simulink model "RPF_Mecanum_02"  (R2020b)
settings: Solver=VariableStepAuto  StartTime=0.0  StopTime=300  MaxStep=0.1  RelTol=1e-3
InitFcn:
  | RadioRueda = 0.05;
  | l1 = 0.15;
  | l2 = 0.15;
libraries: dspsigops x1, simulink x1
settings Model: Creator=rpiza  LastModifiedBy=Racarla

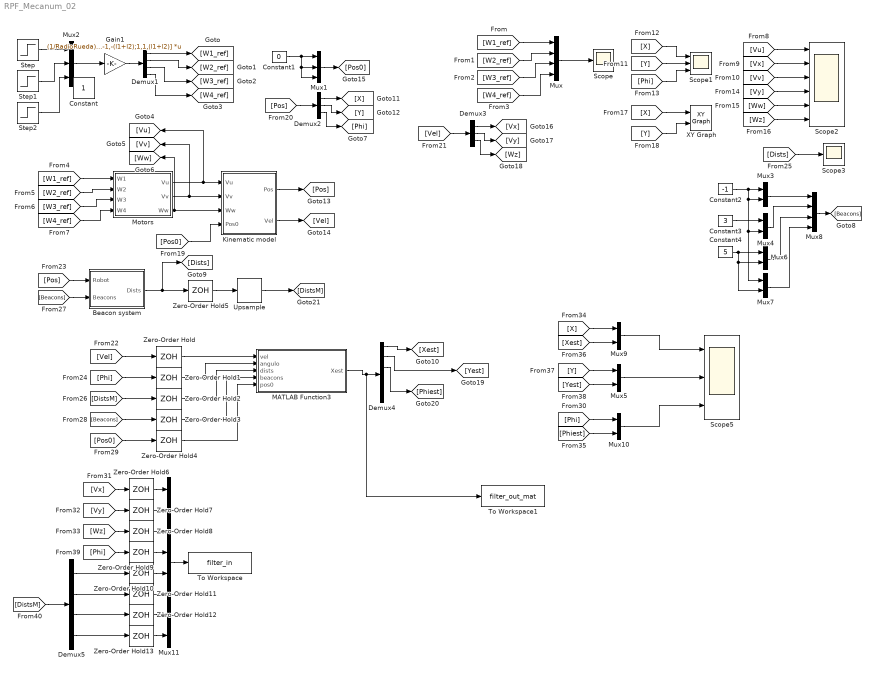
== system RPF_Mecanum_02 ==
  Beacon system : Subsystem
  Constant1 : Constant  Value=0
  Constant2 : Constant  Value=-1
  Constant3 : Constant  Value=3
  Constant4 : Constant  Value=5
  Demux1 : Demux
  Demux2 : Demux  Outputs=3
  Demux3 : Demux  Outputs=3
  Demux4 : Demux  Outputs=6
  Demux5 : Demux
  Gain1 : Gain  Gain=(1/RadioRueda)*[1,1,-(l1+l2); 1,-1,(l1+l2);1,-1,-(l1+l2);1,1,(l1+l2)]  Multiplication=Matrix(K*u) (u vector)
  Kinematic model : Subsystem
  MATLAB Function3 : MATLAB Function  TreatAsAtomicUnit=on
  Motors : Subsystem
  Mux : Mux
  Mux1 : Mux  Inputs=3
  Mux{3..7,9..10} (7 alike) : Mux  Inputs=2
  Mux11 : Mux  Inputs=8
  Mux2 : Mux  Inputs=3
  Mux8 : Mux
  Scope : Scope
  Scope1 : Scope  NumInputPorts=3
  Scope2 : Scope  NumInputPorts=6
  Scope3 : Scope
  Scope5 : Scope  NumInputPorts=3
  Step : Step  Time=0  After=0.1  SampleTime=0
  Step1 : Step  Time=5  Before=0.1  After=0  SampleTime=0
  Step2 : Step  Time=10  After=0.05  SampleTime=0
  To Workspace : ToWorkspace  VariableName=filter_in  SaveFormat=Timeseries  SampleTime=-1
  To Workspace1 : ToWorkspace  VariableName=filter_out_mat  SaveFormat=Timeseries  SampleTime=-1
  Upsample : dspsigops/Upsample  N=10  phase=0  RateOptions=Allow multirate processing  ic=0  mode=Unused parameter value
  XY Graph : simulink/Sinks/XY Graph  xmin=-1  xmax=3  ymin=-1  ymax=5  st=-1
  Zero-Order Hold{,1..4,6..13} (13 alike) : ZeroOrderHold  SampleTime=0.1
  Zero-Order Hold5 : ZeroOrderHold
  Constant : Constant  IOType=siggen
  wires:
  [W1_ref] -> Mux/1
  [W2_ref] -> Mux/2
  [W3_ref] -> Mux/3
  [W4_ref] -> Mux/4
  Mux/1 -> Scope/1
  [Vu] -> Scope2/1
  [Vx] -> Scope2/2
  [Vv] -> Scope2/3
  Mux2/1 -> Gain1/1
  [Vy] -> Scope2/4
  [Ww] -> Scope2/5
  [Wz] -> Scope2/6
  Gain1/1 -> Demux1/1
  Step/1 -> Mux2/1
  Step1/1 -> Mux2/2
  Step2/1 -> Mux2/3
  Demux1/1 -> [W1_ref]
  Demux1/4 -> [W4_ref]
  Demux1/3 -> [W3_ref]
  Demux1/2 -> [W2_ref]
  [Y] -> Scope1/2
  [X] -> Scope1/1
  [Phi] -> Scope1/3
  [X] -> XY Graph/1
  [Y] -> XY Graph/2
  Motors/1(Vu) -> [Vu], Kinematic model/1(Vu)
  Motors/2(Vv) -> [Vv], Kinematic model/2(Vv)
  Motors/3(Ww) -> Kinematic model/3(Ww), [Ww]
  [W1_ref] -> Motors/1(W1)
  [W2_ref] -> Motors/2(W2)
  [W3_ref] -> Motors/3(W3)
  [W4_ref] -> Motors/4(W4)
  Kinematic model/1(Pos) -> [Pos]
  Kinematic model/2(Vel) -> [Vel]
  Mux1/1 -> [Pos0]
  [Pos0] -> Kinematic model/4(Pos0)
  Constant1/1 -> Mux1/2, Mux1/3, Mux1/1
  [Pos] -> Demux2/1
  Demux2/1 -> [X]
  Demux2/2 -> [Y]
  Demux2/3 -> [Phi]
  Demux3/3 -> [Wz]
  Demux3/2 -> [Vy]
  Demux3/1 -> [Vx]
  [Vel] -> Demux3/1
  Constant2/1 -> Mux3/1, Mux4/2, Mux7/1, Mux3/2
  Mux3/1 -> Mux8/1
  Constant3/1 -> Mux4/1
  Mux4/1 -> Mux8/2
  Constant4/1 -> Mux6/1, Mux6/2, Mux7/2
  Mux6/1 -> Mux8/3
  Mux7/1 -> Mux8/4
  Mux8/1 -> [Beacons]
  [Pos] -> Beacon system/1(Robot)
  [Beacons] -> Beacon system/2(Beacons)
  Beacon system/1(Dists) -> Zero-Order Hold5/1, [Dists]
  [Dists] -> Scope3/1
  [Vel] -> Zero-Order Hold/1
  [Phi] -> Zero-Order Hold1/1
  [DistsM] -> Zero-Order Hold2/1
  Zero-Order Hold/1 -> MATLAB Function3/1(vel)
  MATLAB Function3/1(Xest) -> To Workspace1/1, Demux4/1
  [Beacons] -> Zero-Order Hold3/1
  Zero-Order Hold1/1 -> MATLAB Function3/2(angulo)
  Zero-Order Hold2/1 -> MATLAB Function3/3(dists)
  Zero-Order Hold3/1 -> MATLAB Function3/4(beacons)
  [Pos0] -> Zero-Order Hold4/1
  Zero-Order Hold4/1 -> MATLAB Function3/5(pos0)
  Mux5/1 -> Scope5/2
  [X] -> Mux9/1
  [Xest] -> Mux9/2
  Mux9/1 -> Scope5/1
  Demux4/1 -> [Xest]
  Demux4/2 -> [Yest]
  [Yest] -> Mux5/2
  [Y] -> Mux5/1
  [Phi] -> Mux10/1
  [Phiest] -> Mux10/2
  Demux4/3 -> [Phiest]
  Mux10/1 -> Scope5/3
  Zero-Order Hold5/1 -> Upsample/1
  Upsample/1 -> [DistsM]
  Mux11/1 -> To Workspace/1
  Zero-Order Hold6/1 -> Mux11/1
  Zero-Order Hold7/1 -> Mux11/2
  Zero-Order Hold8/1 -> Mux11/3
  Zero-Order Hold9/1 -> Mux11/4
  Zero-Order Hold10/1 -> Mux11/5
  Zero-Order Hold11/1 -> Mux11/6
  Zero-Order Hold12/1 -> Mux11/7
  Zero-Order Hold13/1 -> Mux11/8
  [Vx] -> Zero-Order Hold6/1
  [Vy] -> Zero-Order Hold7/1
  [Wz] -> Zero-Order Hold8/1
  [Phi] -> Zero-Order Hold9/1
  Demux5/1 -> Zero-Order Hold10/1
  Demux5/2 -> Zero-Order Hold11/1
  Demux5/3 -> Zero-Order Hold12/1
  Demux5/4 -> Zero-Order Hold13/1
  [DistsM] -> Demux5/1

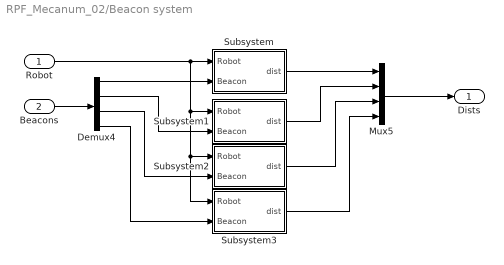
== system RPF_Mecanum_02/Beacon system ==
  Robot : Inport
  Beacons : Inport  Port=2
  Demux4 : Demux
  Mux5 : Mux
  Subsystem : Subsystem
  Subsystem1 : Subsystem
  Subsystem2 : Subsystem
  Subsystem3 : Subsystem
  Dists : Outport
  wires:
  Subsystem/1(dist) -> Mux5/1
  Mux5/1 -> Dists/1
  Robot/1 -> Subsystem/1(Robot), Subsystem1/1(Robot), Subsystem2/1(Robot), Subsystem3/1(Robot)
  Subsystem2/1(dist) -> Mux5/3
  Beacons/1 -> Demux4/1
  Subsystem1/1(dist) -> Mux5/2
  Subsystem3/1(dist) -> Mux5/4
  Demux4/1 -> Subsystem/2(Beacon)
  Demux4/2 -> Subsystem1/2(Beacon)
  Demux4/3 -> Subsystem2/2(Beacon)
  Demux4/4 -> Subsystem3/2(Beacon)

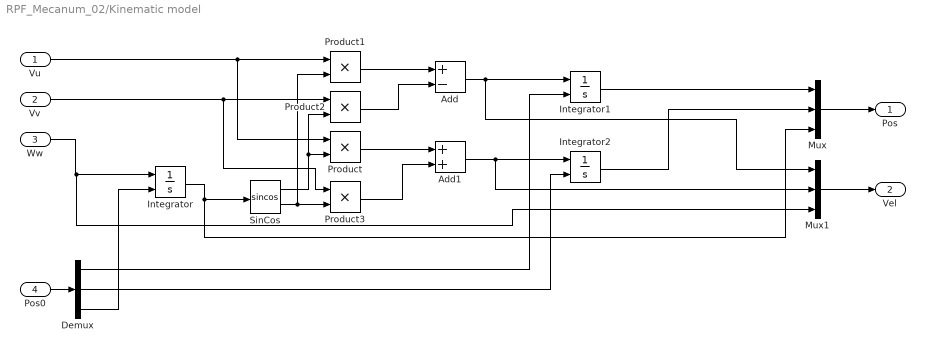
== system RPF_Mecanum_02/Kinematic model ==
  Vu : Inport
  Vv : Inport  Port=2
  Ww : Inport  Port=3
  Pos0 : Inport  Port=4
  Add : Sum  Inputs=+-
  Add1 : Sum
  Demux : Demux  Outputs=3
  Integrator : Integrator  InitialConditionSource=external
  Integrator1 : Integrator  InitialConditionSource=external
  Integrator2 : Integrator  InitialConditionSource=external
  Mux : Mux  Inputs=3
  Mux1 : Mux  Inputs=3
  Product{,1..3} (4 alike) : Product
  SinCos : Trigonometry  Operator=sincos
  Pos : Outport
  Vel : Outport  Port=2
  wires:
  Product/1 -> Add1/1
  SinCos/2 -> Product3/2, Product1/2
  Vv/1 -> Product3/1, Product2/1
  Add1/1 -> Mux1/2, Integrator2/1
  Ww/1 -> Mux1/3, Integrator/1
  Product2/1 -> Add/2
  Add/1 -> Mux1/1, Integrator1/1
  SinCos/1 -> Product2/2, Product/2
  Product3/1 -> Add1/2
  Integrator/1 -> Mux/3, SinCos/1
  Vu/1 -> Product/1, Product1/1
  Product1/1 -> Add/1
  Integrator2/1 -> Mux/2
  Integrator1/1 -> Mux/1
  Mux/1 -> Pos/1
  Mux1/1 -> Vel/1
  Pos0/1 -> Demux/1
  Demux/1 -> Integrator1/2
  Demux/2 -> Integrator2/2
  Demux/3 -> Integrator/2

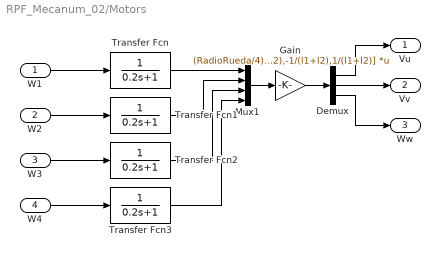
== system RPF_Mecanum_02/Motors ==
  W1 : Inport
  W2 : Inport  Port=2
  W3 : Inport  Port=3
  W4 : Inport  Port=4
  Demux : Demux  Outputs=3
  Gain : Gain  Gain=(RadioRueda/4)*[1,1,1,1;1,-1,-1,1;-1/(l1+l2),1/(l1+l2),-1/(l1+l2),1/(l1+l2)]  Multiplication=Matrix(K*u) (u vector)
  Mux1 : Mux
  Transfer Fcn{,1..3} (4 alike) : TransferFcn  Denominator=[0.2 1]
  Vu : Outport
  Vv : Outport  Port=2
  Ww : Outport  Port=3
  wires:
  Demux/2 -> Vv/1
  Mux1/1 -> Gain/1
  Transfer Fcn2/1 -> Mux1/3
  W4/1 -> Transfer Fcn3/1
  Transfer Fcn1/1 -> Mux1/2
  W3/1 -> Transfer Fcn2/1
  Transfer Fcn/1 -> Mux1/1
  Transfer Fcn3/1 -> Mux1/4
  Gain/1 -> Demux/1
  W2/1 -> Transfer Fcn1/1
  Demux/1 -> Vu/1
  W1/1 -> Transfer Fcn/1
  Demux/3 -> Ww/1

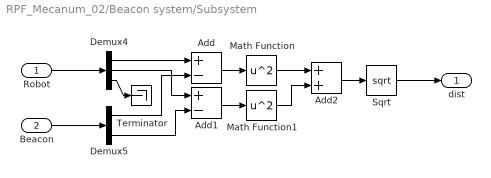
== system RPF_Mecanum_02/Beacon system/Subsystem ==
  Robot : Inport
  Beacon : Inport  Port=2
  Add : Sum  Inputs=+-
  Add1 : Sum  Inputs=+-
  Add2 : Sum
  Demux4 : Demux  Outputs=3
  Demux5 : Demux  Outputs=2
  Math Function : Math  Operator=square  SaturateOnIntegerOverflow=on
  Math Function1 : Math  Operator=square  SaturateOnIntegerOverflow=on
  Sqrt : Sqrt  SaturateOnIntegerOverflow=on
  Terminator : Terminator
  dist : Outport
  wires:
  Math Function/1 -> Add2/1
  Demux4/3 -> Terminator/1
  Add1/1 -> Math Function1/1
  Demux4/1 -> Add/1
  Math Function1/1 -> Add2/2
  Demux4/2 -> Add1/1
  Add/1 -> Math Function/1
  Robot/1 -> Demux4/1
  Add2/1 -> Sqrt/1
  Demux5/2 -> Add1/2
  Demux5/1 -> Add/2
  Beacon/1 -> Demux5/1
  Sqrt/1 -> dist/1

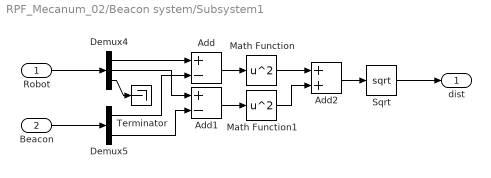
== system RPF_Mecanum_02/Beacon system/Subsystem1 ==
  Robot : Inport
  Beacon : Inport  Port=2
  Add : Sum  Inputs=+-
  Add1 : Sum  Inputs=+-
  Add2 : Sum
  Demux4 : Demux  Outputs=3
  Demux5 : Demux  Outputs=2
  Math Function : Math  Operator=square  SaturateOnIntegerOverflow=on
  Math Function1 : Math  Operator=square  SaturateOnIntegerOverflow=on
  Sqrt : Sqrt  SaturateOnIntegerOverflow=on
  Terminator : Terminator
  dist : Outport
  wires:
  Sqrt/1 -> dist/1
  Beacon/1 -> Demux5/1
  Demux5/1 -> Add/2
  Demux5/2 -> Add1/2
  Add2/1 -> Sqrt/1
  Robot/1 -> Demux4/1
  Add/1 -> Math Function/1
  Demux4/2 -> Add1/1
  Math Function1/1 -> Add2/2
  Demux4/1 -> Add/1
  Add1/1 -> Math Function1/1
  Demux4/3 -> Terminator/1
  Math Function/1 -> Add2/1

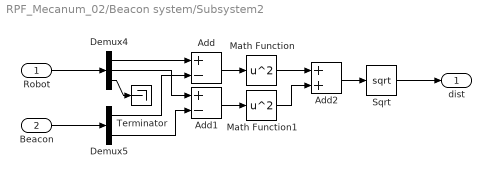
== system RPF_Mecanum_02/Beacon system/Subsystem2 ==
  Robot : Inport
  Beacon : Inport  Port=2
  Add : Sum  Inputs=+-
  Add1 : Sum  Inputs=+-
  Add2 : Sum
  Demux4 : Demux  Outputs=3
  Demux5 : Demux  Outputs=2
  Math Function : Math  Operator=square  SaturateOnIntegerOverflow=on
  Math Function1 : Math  Operator=square  SaturateOnIntegerOverflow=on
  Sqrt : Sqrt  SaturateOnIntegerOverflow=on
  Terminator : Terminator
  dist : Outport
  wires:
  Math Function/1 -> Add2/1
  Demux4/3 -> Terminator/1
  Add1/1 -> Math Function1/1
  Demux4/1 -> Add/1
  Math Function1/1 -> Add2/2
  Demux4/2 -> Add1/1
  Add/1 -> Math Function/1
  Robot/1 -> Demux4/1
  Add2/1 -> Sqrt/1
  Demux5/2 -> Add1/2
  Demux5/1 -> Add/2
  Beacon/1 -> Demux5/1
  Sqrt/1 -> dist/1

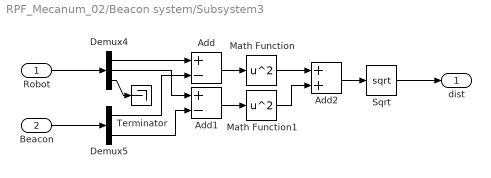
== system RPF_Mecanum_02/Beacon system/Subsystem3 ==
  Robot : Inport
  Beacon : Inport  Port=2
  Add : Sum  Inputs=+-
  Add1 : Sum  Inputs=+-
  Add2 : Sum
  Demux4 : Demux  Outputs=3
  Demux5 : Demux  Outputs=2
  Math Function : Math  Operator=square  SaturateOnIntegerOverflow=on
  Math Function1 : Math  Operator=square  SaturateOnIntegerOverflow=on
  Sqrt : Sqrt  SaturateOnIntegerOverflow=on
  Terminator : Terminator
  dist : Outport
  wires:
  Sqrt/1 -> dist/1
  Beacon/1 -> Demux5/1
  Demux5/1 -> Add/2
  Demux5/2 -> Add1/2
  Add2/1 -> Sqrt/1
  Robot/1 -> Demux4/1
  Add/1 -> Math Function/1
  Demux4/2 -> Add1/1
  Math Function1/1 -> Add2/2
  Demux4/1 -> Add/1
  Add1/1 -> Math Function1/1
  Demux4/3 -> Terminator/1
  Math Function/1 -> Add2/1

== matlab function RPF_Mecanum_02/MATLAB Function3 ==
  data: vel input; Xest output; angulo input; dists input; beacons input; pos0 input
function Xest = EKalman2(vel, angulo, dists, beacons, pos0) %(distancias,velocidad,angulo,posiciones)

%Declaración e inicialización de variables persistentes
%Persisten de un muestreo al siguiente
persistent P;
persistent X;

if isempty(P)
    P = zeros(14, 14); %Se añaden 8 estados para las retenciones de medidas Vu, Vv, Wz, ang, d1, d2, d3, d4
    X = [pos0(1); pos0(2); pos0(3); zeros(3,1); zeros(8, 1)];
else
    delta1 = 1; delta2 = 1; delta3 = 1; delta4 = 1; %Siempre hay medidas de odometría y ángulo
    DBaliza1 = dists(1);  DBaliza2 = dists(2); DBaliza3 = dists(3);  DBaliza4 = dists(4);
    if DBaliza1 == 0 delta5 = 0; else delta5 = 1; end
    if DBaliza2 == 0 delta6 = 0; else delta6 = 1; end
    if DBaliza3 == 0 delta7 = 0; else delta7 = 1; end
    if DBaliza4 == 0 delta8 = 0; else delta8 = 1; end
    Delta = diag([delta1, delta2, delta3, delta4, delta5, delta6, delta7, delta8]);
    PosBaliza1x = beacons(1); PosBaliza1y = beacons(2);
    PosBaliza2x = beacons(3); PosBaliza2y = beacons(4);
    PosBaliza3x = beacons(5); PosBaliza3y = beacons(6);
    PosBaliza4x = beacons(7); PosBaliza4y = beacons(8);
    Vumedida = vel(1); Vvmedida = vel(2); Wwmedida = vel(3);
    
    %Declaración de variables normales
    Ts = 0.1; %Periodo rápido filtro monofrecuencia
    x = X(1); y = X(2); phi = X(3); Vu = X(4); Vv = X(5); Wz = X(6);
    nu1 = X(7); nu2 = X(8); nu3 = X(9); nu4 = X(10); nu5 = X(11);
    nu6 = X(12); nu7 = X(13); nu8 = X(14);
    
    %Matrices del sistema
    % 8x1
%     gkSR = [Vu; 
%         Vv; 
%         Wz; 
%         phi;
%         sqrt((x-PosBaliza1x)^2 + (y-PosBaliza1y)^2);
%         sqrt((x-PosBaliza2x)^2 + (y-PosBaliza2y)^2);
%         sqrt((x-PosBaliza3x)^2 + (y-PosBaliza3y)^2);
%         sqrt((x-PosBaliza4x)^2 + (y-PosBaliza4y)^2)];
    %gk = Delta*gkSR + (eye(8)-Delta)*[nu1; nu2; nu3; nu4; nu5; nu6; nu7; nu8];
    
    % Varianzas estimadas
    Q = diag([30, 30, 30]);
    R = diag([1e-1, 1e-1, 1e-1, 1e-5, 1e-5, 1e-5, 1e-5, 1e-5]);
    z = [Vumedida; Vvmedida; Wwmedida; angulo; DBaliza1; DBaliza2; DBaliza3; DBaliza4];
    
    % 6x3
    HkSR = [((Ts^2)/2)*cos(phi), -((Ts^2)/2)*sin(phi), 0;
        ((Ts^2)/2)*sin(phi), ((Ts^2)/2)*cos(phi), 0; 
        0, 0, (Ts^2)/2;
        Ts, 0, 0; 
        0, Ts, 0; 
        0, 0, Ts];
    Hk = [HkSR; zeros(8,3)]; % (6+8)=14x3
    
    % 8x6
    dgkSR = [
        0, 0, 0, 1, 0, 0;
        0, 0, 0, 0, 1, 0;
        0, 0, 0, 0, 0, 1;
        0, 0, 1, 0, 0, 0;
        (x-PosBaliza1x)/sqrt((x-PosBaliza1x)^2 + (y-PosBaliza1y)^2), (y-PosBaliza1y)/sqrt((x-PosBaliza1x)^2 + (y-PosBaliza1y)^2), 0, 0, 0, 0;
        (x-PosBaliza2x)/sqrt((x-PosBaliza2x)^2 + (y-PosBaliza2y)^2), (y-PosBaliza2y)/sqrt((x-PosBaliza2x)^2 + (y-PosBaliza2y)^2), 0, 0, 0, 0;
        (x-PosBaliza3x)/sqrt((x-PosBaliza3x)^2 + (y-PosBaliza3y)^2), (y-PosBaliza3y)/sqrt((x-PosBaliza3x)^2 + (y-PosBaliza3y)^2), 0, 0, 0, 0;
        (x-PosBaliza4x)/sqrt((x-PosBaliza4x)^2 + (y-PosBaliza4y)^2), (y-PosBaliza4y)/sqrt((x-PosBaliza4x)^2 + (y-PosBaliza4y)^2), 0, 0, 0, 0];    
    % 6x6
    dfkSR = [1, 0, -Ts*(sin(phi)*Vu+cos(phi)*Vv), Ts*cos(phi), -Ts*sin(phi), 0;
        0, 1, Ts*(cos(phi)*Vu-sin(phi)*Vv), Ts*sin(phi), Ts*cos(phi),0;
        0, 0, 1, 0, 0, Ts; 
        0, 0, 0, 1, 0, 0;
        0, 0, 0, 0, 1, 0; 
        0, 0, 0, 0, 0, 1];
    dfk = [dfkSR, zeros(6,8); Delta*dgkSR, eye(8)-Delta];
    dgk = [Delta*dgkSR, eye(8)-Delta]; % 8x16
    
    
    P = dfk*P*dfk' + Hk*Q*Hk';
    
    K = P*dgk'*inv(dgk*P*dgk' + R)*Delta;
    
    P = P - K*dgk*P;
    
    X = [x+Ts*(Vu*cos(phi)-Vv*sin(phi)); y+Ts*(Vu*sin(phi)-Vv*cos(phi)); phi+Ts*Wz; Vu; Vv; Wz;
        delta1*Vu + (1-delta1)*nu1; delta2*Vv + (1-delta2)*nu2; delta3*Wz + (1-delta3)*nu3;
        delta4*phi + (1-delta4)*nu4;
        delta5*sqrt((x-PosBaliza1x)^2 + (y-PosBaliza1y)^2)+(1-delta5)*nu5;
        delta6*sqrt((x-PosBaliza2x)^2 + (y-PosBaliza2y)^2)+(1-delta6)*nu6;
        delta7*sqrt((x-PosBaliza3x)^2 + (y-PosBaliza3y)^2)+(1-delta7)*nu7;
        delta8*sqrt((x-PosBaliza4x)^2 + (y-PosBaliza4y)^2)+(1-delta8)*nu8];
    
    x = X(1); y = X(2); phi = X(3); Vu = X(4); Vv = X(5); Wz = X(6);
    
    nu1 = X(7); nu2 = X(8); nu3 = X(9); nu4 = X(10); nu5 = X(11);
    nu6 = X(12); nu7 = X(13); nu8 = X(14);
    
    gkSR = [Vu; Vv; Wz; phi;
        sqrt((x-PosBaliza1x)^2 + (y-PosBaliza1y)^2);
        sqrt((x-PosBaliza2x)^2 + (y-PosBaliza2y)^2);
        sqrt((x-PosBaliza3x)^2 + (y-PosBaliza3y)^2);
        sqrt((x-PosBaliza4x)^2 + (y-PosBaliza4y)^2)];
    
    gk = Delta*gkSR + (eye(8)-Delta)*[nu1; nu2; nu3; nu4; nu5; nu6; nu7; nu8];
    
    X = X + K*(z - gk);
end
Xest = X(1:6);
